simulink model "LCK_old"  (R2018b)
settings: Solver=FixedStepDiscrete  StartTime=0.0  StopTime=inf  FixedStep=0.005  RelTol=1e-3
PostLoadFcn:
  | if any(exist('dsrtsu_mdlpostloadfcn', 'file') ~= 0), dsrtsu_mdlpostloadfcn('Execute', bdroot); end
values from neighbouring files (symbols this model uses):
  C_DEG2RAD = 0.0175    [LCK_Macro.sldd]
  C_KPH2MPS = 0.2778    [LCK_Macro.sldd]
  C_NEARZERO = 0.0001    [LCK_Macro.sldd]
  C_ONE = 1.0    [LCK_Macro.sldd]
  C_RAD2DEG = 57.2958    [LCK_Macro.sldd]
  C_ZERO = 0.0    [LCK_Macro.sldd]
  k_accel_pedal_pos_per_speed_x : value not decoded    [LCK_LogicPara.sldd]
  k_accel_pedal_pos_per_speed_z : value not decoded    [LCK_LogicPara.sldd]
  k_brake_suprress_hold = 1000.0    [LCK_LogicPara.sldd]
  k_driver_appl_torque_filt = 50.0    [LCK_LogicPara.sldd]
  k_driver_suppression_hold_time = 3000.0    [LCK_LogicPara.sldd]
  k_hands_on_wheel_hold_msec = 500.0    [LCK_LogicPara.sldd]
  k_hands_on_wheel_torque_hi = 0.2    [LCK_LogicPara.sldd]
  k_hands_on_wheel_torque_lo = 0.15    [LCK_LogicPara.sldd]
  k_handsoff_delay_cycles = 50.0    [LCK_LogicPara.sldd]
  k_handsoff_torq_Lo_CR = 0.3    [LCK_LogicPara.sldd]
  k_handson_delay_cycles = 5.0    [LCK_LogicPara.sldd]
  k_HighAccel_suppress_hold = 3000.0    [LCK_LogicPara.sldd]
  k_HLR_suprress_hold = 3000.0    [LCK_LogicPara.sldd]
  k_hs_StrAng_CR_threshold_z : value not decoded    [LCK_LogicPara.sldd]
  k_LC_Exit_Switch = 0.0    [LCK_LogicPara.sldd]
  k_LCG_Configured = 1.0    [LCK_LogicPara.sldd]
  k_LCK_A0_Rdy2Act_UseConst = 0.0    [LCK_LogicPara.sldd]
  k_LCK_A0Fac_ActSta : value not decoded    [LCK_CtrlPara.sldd]
  k_LCK_A0Fac_DrvStm : value not decoded    [LCK_CtrlPara.sldd]
  k_LCK_A0Shift_LftCurv : value not decoded    [LCK_CtrlPara.sldd]
  k_LCK_A0Shift_RgtCurv : value not decoded    [LCK_CtrlPara.sldd]
  k_LCK_A0Shift_StraLan = 0.0    [LCK_CtrlPara.sldd]
  k_LCK_A0ShiftFac_Dy_LftCurv : value not decoded    [LCK_CtrlPara.sldd]
  k_LCK_A0ShiftFac_Dy_RgtCurv : value not decoded    [LCK_CtrlPara.sldd]
  k_LCK_A0ShiftFac_Vspd : value not decoded    [LCK_CtrlPara.sldd]
  k_LCK_accel_inhibit_thold = 35.0    [LCK_LogicPara.sldd]
  k_LCK_Active2Ready_Mask = 255.0    [LCK_LogicPara.sldd]
  k_LCK_CvatRateBks : value not decoded    [LCK_CtrlPara.sldd]
  k_LCK_CvatrBks : value not decoded    [LCK_CtrlPara.sldd]
  k_LCK_DFac_Dy : value not decoded    [LCK_CtrlPara.sldd]
  k_LCK_DFac_Dy_Curv : value not decoded    [LCK_CtrlPara.sldd]
  k_LCK_DFac_HaCurCen : value not decoded    [LCK_CtrlPara.sldd]
  k_LCK_DFac_HaCurSid : value not decoded    [LCK_CtrlPara.sldd]
  k_LCK_DFac_HadCurCen : value not decoded    [LCK_CtrlPara.sldd]
  k_LCK_DFac_HadCurSid : value not decoded    [LCK_CtrlPara.sldd]
  k_LCK_DFac_HadStrCen : value not decoded    [LCK_CtrlPara.sldd]
  k_LCK_DFac_HadStrSid : value not decoded    [LCK_CtrlPara.sldd]
  k_LCK_DFac_HaStrCen : value not decoded    [LCK_CtrlPara.sldd]
  k_LCK_DFac_HaStrSid : value not decoded    [LCK_CtrlPara.sldd]
  k_LCK_DFac_Rad : value not decoded    [LCK_CtrlPara.sldd]
  k_LCK_DFac_SA_CurCen : value not decoded    [LCK_CtrlPara.sldd]
  k_LCK_DFac_SA_CurSid : value not decoded    [LCK_CtrlPara.sldd]
  k_LCK_DFac_SA_StrCen : value not decoded    [LCK_CtrlPara.sldd]
  k_LCK_DFac_SA_StrSid : value not decoded    [LCK_CtrlPara.sldd]
  k_LCK_DFac_SS_CurCen : value not decoded    [LCK_CtrlPara.sldd]
  k_LCK_DFac_SS_CurSid : value not decoded    [LCK_CtrlPara.sldd]
  k_LCK_DFac_SS_StrCen : value not decoded    [LCK_CtrlPara.sldd]
  k_LCK_DFac_SS_StrSid : value not decoded    [LCK_CtrlPara.sldd]
  k_LCK_DFac_Vspd : value not decoded    [LCK_CtrlPara.sldd]
  k_LCK_DlyTm_DrvStim = 0.2    [LCK_CtrlPara.sldd]
  k_LCK_DTermMax = 2.0    [LCK_CtrlPara.sldd]
  k_LCK_DyBks_Curv : value not decoded    [LCK_CtrlPara.sldd]
  k_LCK_Enable_POOnly = 1.0    [LCK_LogicPara.sldd]
  k_LCK_Entry_DistBuffer = 0.1    [LCK_LogicPara.sldd]
  k_LCK_Fac_Vspd2RngThr_FalRec = 0.23    [LCK_CtrlPara.sldd]
  k_LCK_Ffw_CvatSwh = 0.0    [LCK_CtrlPara.sldd]
  k_LCK_Ffw_DyBks : value not decoded    [LCK_CtrlPara.sldd]
  k_LCK_Ffw_TimCon_CmdFlt = 0.0    [LCK_CtrlPara.sldd]
  k_LCK_FfwDeltaFac_Rad_Lft : value not decoded    [LCK_CtrlPara.sldd]
  k_LCK_FfwDeltaFac_Rad_Rgt : value not decoded    [LCK_CtrlPara.sldd]
  k_LCK_FfwDeltaFac_Vspd : value not decoded    [LCK_CtrlPara.sldd]
  k_LCK_FfwFac_CvatRate_Lft : value not decoded    [LCK_CtrlPara.sldd]
  k_LCK_FfwFac_CvatRate_Rgt : value not decoded    [LCK_CtrlPara.sldd]
  k_LCK_FfwFac_Dy : value not decoded    [LCK_CtrlPara.sldd]
  k_LCK_FfwFac_Rad_Lft : value not decoded    [LCK_CtrlPara.sldd]
  k_LCK_FfwFac_Rad_Rgt : value not decoded    [LCK_CtrlPara.sldd]
  k_LCK_FfwFac_Vspd : value not decoded    [LCK_CtrlPara.sldd]
  k_LCK_FfwTorq_Cvat : value not decoded    [LCK_CtrlPara.sldd]
  k_LCK_HAFac_ActSta : value not decoded    [LCK_CtrlPara.sldd]
  k_LCK_HAFac_DrvStm : value not decoded    [LCK_CtrlPara.sldd]
  k_LCK_HaloTime = 2000.0    [LCK_LogicPara.sldd]
  k_LCK_HaloTime_Switch = 0.0    [LCK_LogicPara.sldd]
  k_LCK_HARFac_ActSta : value not decoded    [LCK_CtrlPara.sldd]
  k_LCK_HARFac_DrvStm : value not decoded    [LCK_CtrlPara.sldd]
  k_LCK_Hed_DyBks : value not decoded    [LCK_CtrlPara.sldd]
  k_LCK_HedAngDiffX : value not decoded    [LCK_CtrlPara.sldd]
  k_LCK_HedAngRateDiffX : value not decoded    [LCK_CtrlPara.sldd]
  k_LCK_HndsOnWhel_DlyTm_Idl2Rdy = 0.0    [LCK_LogicPara.sldd]
  k_LCK_host_veh_width = 1.86    [LCK_LogicPara.sldd]
  k_LCK_Idle2Ready_Mask = 239.0    [LCK_LogicPara.sldd]
  k_LCK_Junc_SusTime = 1.0    [LCK_LogicPara.sldd]
  k_LCK_KpKdDecSlopeLmt = 10.0    [LCK_CtrlPara.sldd]
  k_LCK_KpKdIncSlopeLmt = 5.0    [LCK_CtrlPara.sldd]
  k_LCK_Lat_Ctrl_DFac_Lft = 1.0    [LCK_CtrlPara.sldd]
  k_LCK_Lat_Ctrl_DFac_Rgt = 1.05    [LCK_CtrlPara.sldd]
  k_LCK_Lat_Ctrl_Kd = 0.8    [LCK_CtrlPara.sldd]
  k_LCK_Lat_Ctrl_Ki = 0.5    [LCK_CtrlPara.sldd]
  k_LCK_Lat_Ctrl_Kp = 0.7    [LCK_CtrlPara.sldd]
  k_LCK_Lat_Ctrl_Kp_NearGain = 0.7    [LCK_CtrlPara.sldd]
  k_LCK_Lat_Ctrl_PFac_Lft = 1.0    [LCK_CtrlPara.sldd]
  k_LCK_Lat_Ctrl_PFac_Rgt = 1.05    [LCK_CtrlPara.sldd]
  k_LCK_Lat_Ctrl_TimCon_CmdFlt = 5.0    [LCK_CtrlPara.sldd]
  k_LCK_Lat_DFac_Rad : value not decoded    [LCK_CtrlPara.sldd]
  k_LCK_Lat_DFac_SS_Cur : value not decoded    [LCK_CtrlPara.sldd]
  k_LCK_Lat_DFac_SS_Str : value not decoded    [LCK_CtrlPara.sldd]
  k_LCK_Lat_DFac_Vspd : value not decoded    [LCK_CtrlPara.sldd]
  k_LCK_Lat_DyBks : value not decoded    [LCK_CtrlPara.sldd]
  k_LCK_Lat_IFac_Rad : value not decoded    [LCK_CtrlPara.sldd]
  k_LCK_Lat_IFac_Vspd : value not decoded    [LCK_CtrlPara.sldd]
  k_LCK_Lat_ILmtFac_Dy_CurvLan : value not decoded    [LCK_CtrlPara.sldd]
  k_LCK_Lat_ILmtFac_Dy_StraLan : value not decoded    [LCK_CtrlPara.sldd]
  k_LCK_Lat_ILmtFac_Rad : value not decoded    [LCK_CtrlPara.sldd]
  k_LCK_Lat_ILmtFac_Rad_NearGain = 1.0    [LCK_CtrlPara.sldd]
  k_LCK_Lat_ILmtFac_Vspd_CurvLan : value not decoded    [LCK_CtrlPara.sldd]
  k_LCK_Lat_ILmtFac_Vspd_StraLan : value not decoded    [LCK_CtrlPara.sldd]
  k_LCK_Lat_ITermLmt_Dy = 1.0    [LCK_CtrlPara.sldd]
  k_LCK_Lat_KpKdDecSlopeLmt = 10.0    [LCK_CtrlPara.sldd]
  k_LCK_Lat_KpKdIncSlopeLmt = 10.0    [LCK_CtrlPara.sldd]
  k_LCK_Lat_PFac_Dy_InnLftCur : value not decoded    [LCK_CtrlPara.sldd]
  k_LCK_Lat_PFac_Dy_InnRgtCur : value not decoded    [LCK_CtrlPara.sldd]
  k_LCK_Lat_PFac_Dy_OutLftCur : value not decoded    [LCK_CtrlPara.sldd]
  k_LCK_Lat_PFac_Dy_OutRgtCur : value not decoded    [LCK_CtrlPara.sldd]
  k_LCK_Lat_PFac_Dy_Str : value not decoded    [LCK_CtrlPara.sldd]
  k_LCK_Lat_PFac_Rad : value not decoded    [LCK_CtrlPara.sldd]
  ... (+158 more)
undefined symbols (not defined in the file or in its folder): k_LCK_CurvBks, K_LCK_SPA0A1A2_LMRngCmp_y
libraries: LateralControl_fcns_lib x58, simulink x22
(part 18 of 45)

== system LCK_old/Lateral_Control_Module/Adas_Lateral_Control_LCK_Core/Module 3/Sig_Wekng_1 ==
  Steer_Torq : Inport
  Abs : Abs  Tag={'output',{'type','Float32'},'date',737464.51221858792}  Description=_GWMH9P4.LCK.000_195_
  Constant1 : Constant  Tag={'output',{'type','Int32'},'date',737462.5090449769}  Description=_GWMH9P4.LCK.000_208_  OutDataTypeStr=single
  Constant2 : Constant  Tag={'output',{'type','Int32'},'date',737462.5090449769}  Description=_GWMH9P4.LCK.000_208_  OutDataTypeStr=single
  Constant22 : Constant  Tag={'output',{'type','Int32'},'date',737462.5090449769}  Description=_GWMH9P4.LCK.000_208_  OutDataTypeStr=single
  Data Type Conversion4 : DataTypeConversion  Description=_GWMH9P4.LCK.000_213_
  Delay_Trig : LateralControl_fcns_lib/Delay_Trig  SystemSampleTime=-1
  Logical Operator : Logic  Operator=OR  AllPortsSameDT=off  OutDataTypeStr=boolean
  Relational Operator : RelationalOperator  Tag={'date',737462.5090511227}  Description=_GWMH9P4.LCK.000_247_  OutDataTypeStr=boolean  RndMeth=Nearest
  Relational Operator6 : RelationalOperator  Tag={'date',737462.5090511227}  Description=_GWMH9P4.LCK.000_247_  Operator=<=  OutDataTypeStr=boolean  RndMeth=Nearest
  Switch1 : Switch  Tag={'output',{'type','Float32'},'threshold',{'type','Int32'},'date',737463.80838512734}  Description=_GWMH9P4.LCK.000_251_  Threshold=0.5
  Switch11 : Switch  Tag={'output',{'type','Float32'},'threshold',{'type','Int32'},'date',737463.80838512734}  Description=_GWMH9P4.LCK.000_251_  Threshold=0.5
  Switch2 : Switch  Tag={'output',{'type','Float32'},'threshold',{'type','Int32'},'date',737463.80838512734}  Description=_GWMH9P4.LCK.000_251_  Threshold=0.5
  Trigger Hold Counter : LateralControl_fcns_lib/Trigger Hold Counter  SystemSampleTime=-1
  k_LCK_A0Fac_DrvStm : Lookup_n-D  Tag={'input',{'name','$P','class','EXTERN_CAL','type','Float32'},'output',{'type','Float32'},'table',{'name','$P','class','EXTERN_CAL','type','Float32'},'date',737534.7265986806}  NumberOfTableDimensions=1  BreakpointsForDimension1=k_LCK_TimBks_DrvStm  IndexSearchMethod=Linear search  Table=k_LCK_A0Fac_DrvStm  ExtrapMethod=Clip  InternalRulePriority=Speed  RndMeth=Simplest  InputSameDT=on
  k_LCK_DlyTm_DrvStim : Constant  Tag={'output',{'name','$P','class','EXTERN_CAL','type','Float32'},'date',737462.72103232634}  Description=_GWMH9P4.LCK.000_268_  Value=k_LCK_DlyTm_DrvStim
  k_LCK_HAFac_DrvStm : Lookup_n-D  Tag={'input',{'name','$P','class','EXTERN_CAL','type','Float32'},'output',{'type','Float32'},'table',{'name','$P','class','EXTERN_CAL','type','Float32'},'date',737534.7265986806}  NumberOfTableDimensions=1  BreakpointsForDimension1=k_LCK_TimBks_DrvStm  IndexSearchMethod=Linear search  Table=k_LCK_HAFac_DrvStm  ExtrapMethod=Clip  InternalRulePriority=Speed  RndMeth=Simplest  InputSameDT=on
  k_LCK_HARFac_DrvStm : Lookup_n-D  Tag={'input',{'name','$P','class','EXTERN_CAL','type','Float32'},'output',{'type','Float32'},'table',{'name','$P','class','EXTERN_CAL','type','Float32'},'date',737534.7265986806}  NumberOfTableDimensions=1  BreakpointsForDimension1=k_LCK_TimBks_DrvStm  IndexSearchMethod=Linear search  Table=k_LCK_HARFac_DrvStm  ExtrapMethod=Clip  InternalRulePriority=Speed  RndMeth=Simplest  InputSameDT=on
  k_LCK_SigFacHldTim_DrvStim : Constant  Tag={'output',{'name','$P','class','EXTERN_CAL','type','Float32'},'date',737532.83577214123}  Description=_GWMH9P4.LCK.000_274_  Value=k_LCK_SigFacHldTim_DrvStim
  k_LCK_TorqThrBig_DrvStim : Constant  Tag={'output',{'name','$P','class','EXTERN_CAL','type','Float32'},'date',737531.64057921292}  Description=_GWMH9P4.LCK.000_273_  Value=k_LCK_TorqThrBig_DrvStim
  k_LCK_TorqThr_DrvStim : Constant  Tag={'output',{'name','$P','class','EXTERN_CAL','type','Float32'},'date',737531.64057921292}  Description=_GWMH9P4.LCK.000_273_  Value=k_LCK_TorqThr_DrvStim
  Drv_Stm_Flag_Held : Outport
  A0Fac_DrvStm : Outport  Port=2
  HAFac_DrvStm : Outport  Port=3
  HARFac_DrvStm : Outport  Port=4
  wires:
  Constant2/1 -> Switch2/3
  k_LCK_SigFacHldTim_DrvStim/1 -> Trigger Hold Counter/2
  Constant1/1 -> Switch1/3
  Switch1/1 -> HAFac_DrvStm/1
  k_LCK_A0Fac_DrvStm/1 -> Switch11/1
  Switch2/1 -> HARFac_DrvStm/1
  k_LCK_HAFac_DrvStm/1 -> Switch1/1
  k_LCK_HARFac_DrvStm/1 -> Switch2/1
  Constant22/1 -> Switch11/3
  Switch11/1 -> A0Fac_DrvStm/1
  Trigger Hold Counter/1 -> Switch2/2, Drv_Stm_Flag_Held/1, Switch1/2, Switch11/2
  Trigger Hold Counter/2 -> k_LCK_HARFac_DrvStm/1, k_LCK_A0Fac_DrvStm/1, k_LCK_HAFac_DrvStm/1
  Logical Operator/1 -> Trigger Hold Counter/1
  Abs/1 -> Relational Operator6/2, Relational Operator/1
  k_LCK_DlyTm_DrvStim/1 -> Delay_Trig/2
  Data Type Conversion4/1 -> Delay_Trig/1
  Relational Operator6/1 -> Data Type Conversion4/1
  Steer_Torq/1 -> Abs/1
  k_LCK_TorqThrBig_DrvStim/1 -> Relational Operator/2
  Delay_Trig/1 -> Logical Operator/1
  Relational Operator/1 -> Logical Operator/2
  k_LCK_TorqThr_DrvStim/1 -> Relational Operator6/1

== system LCK_old/Lateral_Control_Module/Adas_Lateral_Control_LCK_Core/Module 6/Determination Of Cen Flag ==
  Str_Flag : Inport
  Dy_0 : Inport  Port=2
  Abs : Abs
  CenLowLmt0 : Constant  Value=0.2  OutDataTypeStr=single
  CenLowLmt1 : Constant  Value=0.25  OutDataTypeStr=single
  CenUpLmt0 : Constant  Value=0.3  OutDataTypeStr=single
  CenUpLmt1 : Constant  Value=0.35  OutDataTypeStr=single
  Chart : Stateflow chart  TreatAsAtomicUnit=on
  Switch2 : Switch  Description=_GWMAB30P4.LKA.000_512_  Criteria=u2 > Threshold
  Switch5 : Switch  Description=_GWMAB30P4.LKA.000_512_  Criteria=u2 > Threshold
  Cen_Flag : Outport
  wires:
  Dy_0/1 -> Abs/1
  CenUpLmt1/1 -> Switch5/3
  Switch5/1 -> Chart/2(CenUpLmt)
  Abs/1 -> Chart/1(Dy)
  Switch2/1 -> Chart/3(CenLowLmt)
  CenUpLmt0/1 -> Switch5/1
  CenLowLmt1/1 -> Switch2/3
  Str_Flag/1 -> Switch2/2, Switch5/2
  CenLowLmt0/1 -> Switch2/1
  Chart/1(Cen_Flag) -> Cen_Flag/1

== system LCK_old/Lateral_Control_Module/Adas_Lateral_Control_LCK_Core/Module 6/Determination of Str Flag ==
  Road_Radius : Inport
  Chart1 : Stateflow chart  TreatAsAtomicUnit=on
  RadLowLmt : Constant  Value=3800
  RadUpLmt : Constant  Value=4000
  Str_Flag : Outport
  wires:
  RadUpLmt/1 -> Chart1/2(RadiusUpLmt)
  Road_Radius/1 -> Chart1/1(Radius)
  RadLowLmt/1 -> Chart1/3(RadiusLowLmt)
  Chart1/1(Str_Flag) -> Str_Flag/1

== system LCK_old/Lateral_Control_Module/Adas_Lateral_Control_LCK_Core/Module 6/Recognition of Curve Information ==
  Dy_0 : Inport
  Dy_1 : Inport  Port=2
  Curvature_0 : Inport  Port=3
  Compare To Zero : simulink/Logic and Bit Operations/Compare To Zero  relop=<=  OutDataTypeStr=boolean
  Compare To Zero1 : simulink/Logic and Bit Operations/Compare To Zero  relop=>  OutDataTypeStr=boolean
  Compare To Zero2 : simulink/Logic and Bit Operations/Compare To Zero  relop=<  OutDataTypeStr=boolean
  Compare To Zero3 : simulink/Logic and Bit Operations/Compare To Zero  relop=>  OutDataTypeStr=boolean
  Compare To Zero4 : simulink/Logic and Bit Operations/Compare To Zero  relop=<  OutDataTypeStr=boolean
  Relay : Relay  OnSwitchValue=0.02  OffSwitchValue=-0.02  OffOutputValue=-1
  Relay1 : Relay  OnSwitchValue=0.02  OffSwitchValue=-0.02  OffOutputValue=-1
  Switch6 : Switch  Criteria=u2 > Threshold
  Switch7 : Switch  Criteria=u2 > Threshold
  Inn_Cur_Flag_1 : Outport
  Inn_Cur_Flag_0 : Outport  Port=2
  Cur_Lan_Flag : Outport  Port=3
  wires:
  Dy_1/1 -> Relay/1
  Curvature_0/1 -> Compare To Zero/1
  Compare To Zero3/1 -> Switch7/1
  Compare To Zero4/1 -> Switch7/3
  Compare To Zero2/1 -> Switch6/3
  Relay/1 -> Compare To Zero1/1, Compare To Zero2/1
  Relay1/1 -> Compare To Zero3/1, Compare To Zero4/1
  Compare To Zero1/1 -> Switch6/1
  Dy_0/1 -> Relay1/1
  Compare To Zero/1 -> Cur_Lan_Flag/1, Switch7/2, Switch6/2
  Switch6/1 -> Inn_Cur_Flag_1/1
  Switch7/1 -> Inn_Cur_Flag_0/1
